simulink model "gm_sampleModel1512_5_sub"  (R2023a)
settings: Solver=VariableStepAuto  StartTime=0.0  StopTime=10.0  RelTol=1e-3
libraries: simulink x2
settings Model: Creator=user1  LastModifiedBy=user1
settings OptimizationCC: BlockReduction=off  ConditionallyExecuteInputs=off
settings DebuggingCC: InheritedTsInSrcMsg=none

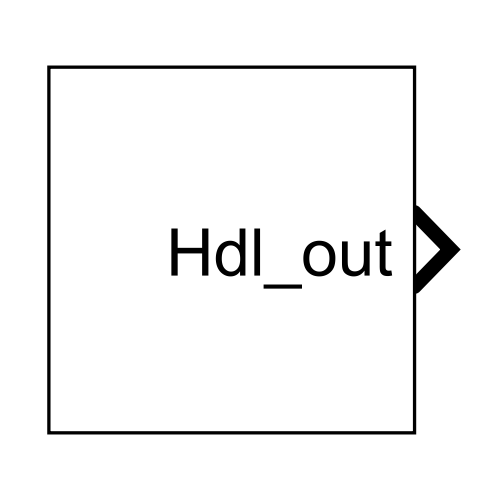
[thumbnail: Simulink's stored preview of the top-level diagram]
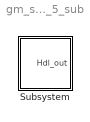
== system gm_sampleModel1512_5_sub ==
  Subsystem : Subsystem

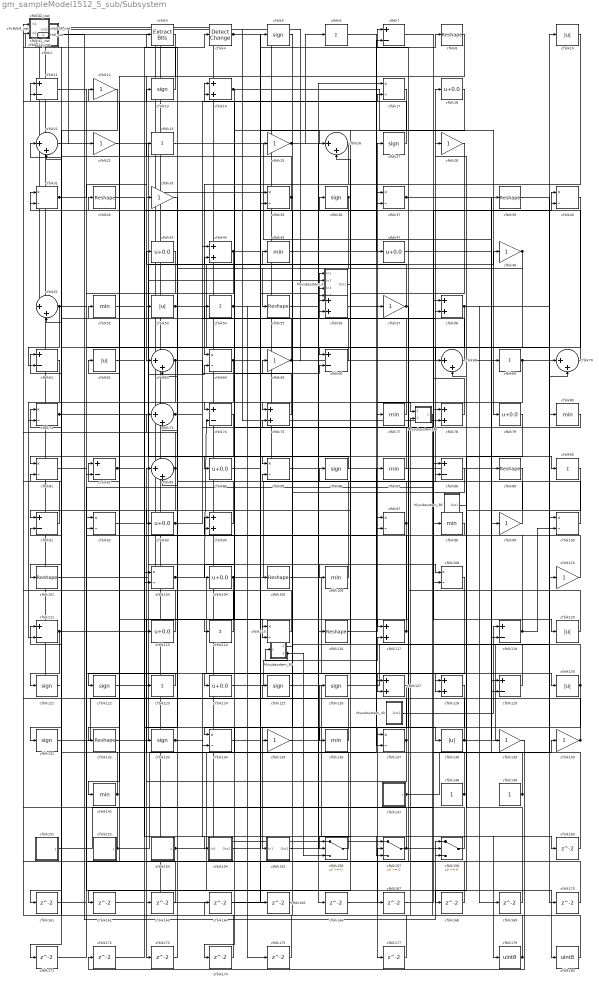
== system gm_sampleModel1512_5_sub/Subsystem ==
  Mysubsystem_3 : Subsystem
  Mysubsystem_30 : Subsystem
  Mysubsystem_36 : Subsystem
  Mysubsystem_38 : Subsystem
  Mysubsystem_40 : Subsystem
  cfblk1 : Subsystem  mask(Detect Rise Nonnegative){vinit=double(0), InputProcessing=Elements as channels (sample based), OutDataTypeStr=uint8}
      mask prompts: vinit "Simulink:masks:InitialCondition_MP"; InputProcessing "Simulink:masks:InputProcessing_MP"; OutDataTypeStr "Simulink:masks:OutputDataType_MP"
      mask help: Simulink:masks:DetectRiseNonnegative_MD
      mask init:
      | InputProcessing = 'Elements as channels (sample based)';
      | OutDataTypeStr = 'uint8';
      | vinit = double(0);
      mask TypeOptions InputProcessing: Simulink:masks:ColumnsAsChannelsFrameBased | Simulink:masks:ElementsAsChannelsSampleBased
      mask TypeOptions OutDataTypeStr: Simulink:masks:uint8 | Simulink:masks:boolean
      mask Display: fprintf('U >= 0\n&  NOT\nU/z >= 0')
  cfblk{10,53,62,120,130,138} (6 alike) : Abs  OutDataTypeStr=uint8  SaturateOnIntegerOverflow=off
  cfblk{17,31,35,37,40,64,71,81,85,92,97,100,103,108,115,134,137} (17 alike) : Product  Inputs=*/  OutDataTypeStr=uint8  RndMeth=Zero  SaturateOnIntegerOverflow=on
  cfblk{8,32,39,55,89,101,105,116,132} (9 alike) : Reshape
  cfblk102_inst : Subsystem
  cfblk{18,43,47,79,84,93,104,113,124} (9 alike) : Bias  Bias=0.0  SaturateOnIntegerOverflow=off
  cfblk{45,52,77,80,87,98,106,136,142} (9 alike) : MinMax  OutDataTypeStr=uint8
  cfblk{7,11,61,66,74,82,88,91,111,119,129} (11 alike) : Sum  Inputs=+-  OutDataTypeStr=uint8
  cfblk{12,22,25,28,33,49,57,65,99,110,135,139..140} (13 alike) : Gain  OutDataTypeStr=uint8
  cfblk112_inst : Subsystem
  cfblk{6,23,54,69,90,114,123} (7 alike) : Sum  Inputs=+  OutDataTypeStr=uint8
  cfblk{14,44,56,58,75,78,94,117,127..128} (10 alike) : Sum  OutDataTypeStr=uint8
  cfblk{5,13,27,36,86,121..122,125..126,131,133} (11 alike) : Signum
  cfblk147 : Subsystem  mask(Counter Free-Running){NumBits=double(16), tsamp=double(-1)}
      mask prompts: NumBits "Simulink:masks:NumberOfBits_MP"; tsamp "Simulink:masks:SampleTime_MP"
      mask help: Simulink:masks:CounterFreeRunning_MD
  cfblk148 : Constant  OutDataTypeStr=uint8  SampleTime=-1
  cfblk149 : Constant  OutDataTypeStr=uint8  SampleTime=-1
  cfblk151 : Subsystem  mask(Counter Free-Running){NumBits=double(16), tsamp=double(-1)}
      mask prompts: NumBits "Simulink:masks:NumberOfBits_MP"; tsamp "Simulink:masks:SampleTime_MP"
      mask help: Simulink:masks:CounterFreeRunning_MD
  cfblk152 : Subsystem  mask(Counter Limited){uplimit=double(7), tsamp=double(-1)}
      mask prompts: uplimit "Simulink:masks:UpperLimit_MP"; tsamp "Simulink:masks:SampleTime_MP"
      mask help: Simulink:masks:CounterLimited_MD
      mask init:
      | nbits = double(8);
      | tsamp = double(-1);
      | uplimit = double(7);
  cfblk153 : Subsystem  mask(Counter Limited){uplimit=double(7), tsamp=double(-1)}
      mask prompts: uplimit "Simulink:masks:UpperLimit_MP"; tsamp "Simulink:masks:SampleTime_MP"
      mask help: Simulink:masks:CounterLimited_MD
      mask init:
      | nbits = double(8);
      | tsamp = double(-1);
      | uplimit = double(7);
  cfblk154 : Subsystem
  cfblk155 : Subsystem
  cfblk156 : Switch  OutDataTypeStr=uint8  SaturateOnIntegerOverflow=off  InputSameDT=off
  cfblk157 : Switch  OutDataTypeStr=uint8  SaturateOnIntegerOverflow=off  InputSameDT=off
  cfblk158 : Switch  OutDataTypeStr=uint8  SaturateOnIntegerOverflow=off  InputSameDT=off
  cfblk{160..175,177} (17 alike) : Delay  SampleTime=1
  cfblk179 : DataTypeConversion  OutDataTypeStr=uint8  SaturateOnIntegerOverflow=off  RndMeth=Floor
  cfblk180 : DataTypeConversion  OutDataTypeStr=uint8  SaturateOnIntegerOverflow=off  RndMeth=Floor
  cfblk2 : Constant  Value=0  OutDataTypeStr=uint8  SampleTime=1
  cfblk{21,26,51,63,68,70,73,83} (8 alike) : Sum  Inputs=|++  OutDataTypeStr=uint8
  cfblk3 : simulink/Logic and Bit Operations/Extract Bits  bitsToExtract=Upper half  numBits=8  bitIdxRange=[0 7]  outScalingMode=Preserve fixed-point scaling
      settings: LibrarySourceBlock=|
      | hdlsllib/Logic and Bit
      | Operations/Extract Bits
  cfblk4 : simulink/Logic and Bit Operations/Detect Change  vinit=0  OutDataTypeStr=uint8
      settings: LibrarySourceBlock=|
      | hdlsllib/Logic and Bit
      | Operations/Detect
      | Change
  cfblk41_inst : Subsystem
  cfblk42_inst : Subsystem
  cfblk59_inst : Subsystem
  cfblk9_inst : Subsystem
  Hdl_out : Outport  OutDataTypeStr=uint8  SampleTime=1
  wires:
  Mysubsystem_3/1(Out1) -> cfblk162/1
  Mysubsystem_30/1(Out1) -> cfblk85/2
  Mysubsystem_30/2(Out2) -> cfblk156/3, cfblk65/1, Mysubsystem_30/1(In1)
  Mysubsystem_36/1(Out1) -> cfblk164/1
  Mysubsystem_38/1(Out1) -> cfblk134/1
  Mysubsystem_40/1(Out1) -> cfblk119/1
  cfblk1/1(Y) -> cfblk158/1
  cfblk10/1 -> cfblk64/1
  cfblk100/1 -> cfblk86/1
  cfblk101/1 -> cfblk108/1
  cfblk102_inst/1(out1) -> cfblk22/1
  cfblk103/1 -> cfblk74/2, cfblk130/1
  cfblk104/1 -> cfblk18/1, cfblk173/1
  cfblk105/1 -> cfblk127/2
  cfblk106/1 -> cfblk42_inst/2(in2)
  cfblk108/1 -> cfblk134/2
  cfblk11/1 -> cfblk92/2
  cfblk110/1 -> Mysubsystem_3/1(In1)
  cfblk111/1 -> cfblk121/1, Mysubsystem_3/2(In2)
  cfblk112_inst/1(out1) -> cfblk9_inst/2(in2), cfblk89/1, cfblk78/2
  cfblk113/1 -> cfblk62/1
  cfblk114/1 -> cfblk102_inst/1(in1)
  cfblk115/1 -> cfblk12/1
  cfblk116/1 -> cfblk27/1
  cfblk117/1 -> cfblk26/2, cfblk77/1
  cfblk119/1 -> cfblk28/1, cfblk100/2
  cfblk12/1 -> cfblk131/1
  cfblk120/1 -> cfblk37/2
  cfblk121/1 -> Hdl_out/1
  cfblk122/1 -> cfblk47/1
  cfblk123/1 -> cfblk122/1
  cfblk124/1 -> cfblk117/2
  cfblk125/1 -> cfblk179/1
  cfblk126/1 -> cfblk80/1
  cfblk127/1 -> cfblk177/1
  cfblk128/1 -> cfblk155/1(In1)
  cfblk129/1 -> cfblk32/1
  cfblk13/1 -> cfblk112_inst/2(in2)
  cfblk130/1 -> cfblk36/1, cfblk174/1, cfblk168/1
  cfblk131/1 -> Mysubsystem_3/3(In3)
  cfblk132/1 -> cfblk64/2
  cfblk133/1 -> cfblk83/2, cfblk156/2
  cfblk134/1 -> cfblk165/1
  cfblk135/1 -> cfblk126/1
  cfblk136/1 -> cfblk71/1
  cfblk137/1 -> cfblk51/2, cfblk163/1
  cfblk138/1 -> cfblk70/2, cfblk45/1
  cfblk139/1 -> cfblk172/1
  cfblk14/1 -> cfblk79/1, cfblk74/1
  cfblk140/1 -> cfblk9_inst/1(in1), cfblk88/2
  cfblk142/1 -> cfblk21/1, cfblk81/2
  cfblk147/1(y) -> cfblk39/1, cfblk10/1
  cfblk148/1 -> cfblk94/1, cfblk83/1
  cfblk149/1 -> cfblk94/2, cfblk61/1
  cfblk151/1(y) -> cfblk98/1
  cfblk152/1(y) -> cfblk5/1, cfblk111/1
  cfblk153/1(y) -> cfblk180/1, cfblk87/1
  cfblk154/1(Out1) -> cfblk56/1
  cfblk155/1(Out1) -> Mysubsystem_3/4(In4)
  cfblk156/1 -> cfblk52/1
  cfblk157/1 -> cfblk102_inst/2(in2), cfblk140/1
  cfblk158/1 -> cfblk97/2
  cfblk160/1 -> cfblk44/2
  cfblk161/1 -> cfblk158/3
  cfblk162/1 -> cfblk97/1
  cfblk163/1 -> cfblk82/1
  cfblk164/1 -> cfblk158/2
  cfblk165/1 -> cfblk1/1(U)
  cfblk166/1 -> cfblk157/2
  cfblk167/1 -> cfblk40/1
  cfblk168/1 -> cfblk7/1
  cfblk169/1 -> cfblk68/2
  cfblk17/1 -> cfblk104/1
  cfblk170/1 -> cfblk41_inst/2(in2)
  cfblk171/1 -> cfblk88/1
  cfblk172/1 -> cfblk37/1
  cfblk173/1 -> cfblk73/2
  cfblk174/1 -> cfblk31/1
  cfblk175/1 -> cfblk91/2
  cfblk177/1 -> cfblk59_inst/1(in1)
  cfblk179/1 -> cfblk3/1, Mysubsystem_36/2(In2)
  cfblk18/1 -> cfblk156/1
  cfblk180/1 -> cfblk125/1
  cfblk2/1 -> cfblk157/1
  cfblk21/1 -> cfblk69/1
  cfblk22/1 -> cfblk90/1
  cfblk23/1 -> cfblk139/1
  cfblk25/1 -> cfblk116/1, cfblk6/1
  cfblk26/1 -> cfblk115/2
  cfblk27/1 -> cfblk42_inst/1(in1)
  cfblk28/1 -> cfblk91/1
  cfblk3/1 -> cfblk63/1
  cfblk31/1 -> cfblk33/1, cfblk167/1
  cfblk32/1 -> cfblk154/1(In1)
  cfblk33/1 -> cfblk113/1
  cfblk35/1 -> cfblk11/1, cfblk31/2
  cfblk36/1 -> cfblk93/1, cfblk85/1
  cfblk37/1 -> cfblk129/1, cfblk40/2
  cfblk39/1 -> cfblk100/1
  cfblk4/1 -> cfblk56/2, cfblk26/1, cfblk108/2
  cfblk40/1 -> cfblk68/1
  cfblk41_inst/1(out1) -> cfblk25/1
  cfblk42_inst/1(out1) -> cfblk35/1
  cfblk43/1 -> cfblk53/1
  cfblk44/1 -> cfblk82/2, cfblk8/1
  cfblk45/1 -> cfblk7/2
  cfblk47/1 -> cfblk119/2
  cfblk49/1 -> cfblk55/1, cfblk129/2, cfblk81/1
  cfblk5/1 -> cfblk75/1
  cfblk51/1 -> cfblk61/2, cfblk128/2
  cfblk52/1 -> cfblk66/1
  cfblk53/1 -> cfblk49/1, cfblk110/1
  cfblk54/1 -> cfblk35/2, cfblk175/1
  cfblk55/1 -> cfblk57/1
  cfblk56/1 -> Mysubsystem_36/1(In1)
  cfblk57/1 -> cfblk13/1, cfblk137/1
  cfblk58/1 -> cfblk63/2, cfblk170/1, cfblk169/1, cfblk114/1
  cfblk59_inst/1(out1) -> cfblk51/1, cfblk105/1
  cfblk6/1 -> cfblk138/1
  cfblk61/1 -> cfblk111/2
  cfblk62/1 -> cfblk103/1
  cfblk63/1 -> cfblk66/2, cfblk171/1
  cfblk64/1 -> cfblk161/1, cfblk160/1
  cfblk65/1 -> cfblk157/3, cfblk112_inst/1(in1)
  cfblk66/1 -> cfblk23/1
  cfblk68/1 -> cfblk44/1
  cfblk69/1 -> cfblk117/1, cfblk71/2
  cfblk7/1 -> cfblk120/1
  cfblk70/1 -> cfblk21/2
  cfblk71/1 -> cfblk99/1, cfblk166/1
  cfblk73/1 -> cfblk58/2, cfblk133/1
  cfblk74/1 -> cfblk101/1
  cfblk75/1 -> cfblk54/1
  cfblk77/1 -> cfblk11/2
  cfblk78/1 -> cfblk58/1
  cfblk79/1 -> cfblk128/1
  cfblk8/1 -> cfblk132/1
  cfblk80/1 -> cfblk75/2
  cfblk81/1 -> cfblk124/1
  cfblk82/1 -> cfblk137/2, cfblk115/1
  cfblk83/1 -> cfblk59_inst/2(in2), cfblk103/2, cfblk123/1
  cfblk84/1 -> cfblk106/1
  cfblk85/1 -> cfblk17/1
  cfblk86/1 -> cfblk84/1
  cfblk87/1 -> cfblk14/1
  cfblk88/1 -> cfblk135/1
  cfblk89/1 -> cfblk127/1
  cfblk9_inst/1(out1) -> cfblk70/1
  cfblk90/1 -> cfblk136/1
  cfblk91/1 -> cfblk41_inst/1(in1)
  cfblk92/1 -> cfblk4/1
  cfblk93/1 -> cfblk78/1, cfblk17/2
  cfblk94/1 -> cfblk43/1
  cfblk97/1 -> cfblk73/1, cfblk142/1
  cfblk98/1 -> cfblk92/1
  cfblk99/1 -> cfblk14/2

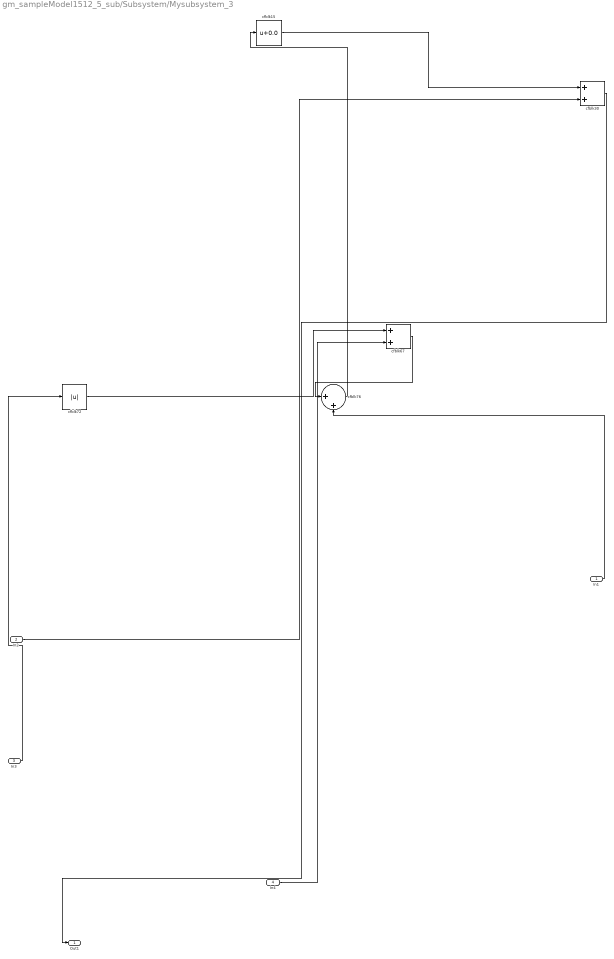
== system gm_sampleModel1512_5_sub/Subsystem/Mysubsystem_3 ==
  In1 : Inport  OutDataTypeStr=uint8  PortDimensions=1  SampleTime=1
  In2 : Inport  Port=2  OutDataTypeStr=uint8  PortDimensions=1  SampleTime=1
  In3 : Inport  Port=3  OutDataTypeStr=uint8  PortDimensions=1  SampleTime=1
  In4 : Inport  Port=4  OutDataTypeStr=uint8  PortDimensions=1  SampleTime=1
  cfblk15 : Bias  Bias=0.0  SaturateOnIntegerOverflow=off
  cfblk30 : Sum
  cfblk67 : Sum
  cfblk72 : Abs  SaturateOnIntegerOverflow=off
  cfblk76 : Sum  Inputs=|++
  Out1 : Outport  SampleTime=1
  wires:
  In1/1 -> cfblk76/2
  In2/1 -> cfblk30/2
  In3/1 -> cfblk72/1
  In4/1 -> cfblk67/2
  cfblk15/1 -> cfblk30/1
  cfblk30/1 -> Out1/1
  cfblk67/1 -> cfblk76/1
  cfblk72/1 -> cfblk67/1
  cfblk76/1 -> cfblk15/1

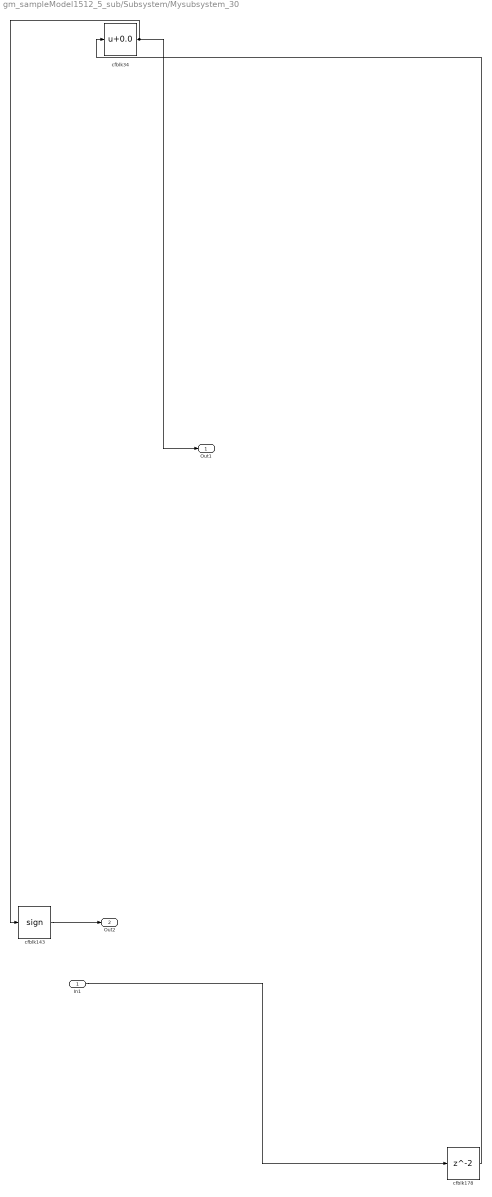
== system gm_sampleModel1512_5_sub/Subsystem/Mysubsystem_30 ==
  In1 : Inport  OutDataTypeStr=uint8  PortDimensions=1  SampleTime=1
  cfblk143 : Signum
  cfblk178 : Delay  SampleTime=1
  cfblk34 : Bias  Bias=0.0  SaturateOnIntegerOverflow=off
  Out1 : Outport  SampleTime=1
  Out2 : Outport  Port=2  SampleTime=1
  wires:
  In1/1 -> cfblk178/1
  cfblk143/1 -> Out2/1
  cfblk178/1 -> cfblk34/1
  cfblk34/1 -> cfblk143/1, Out1/1

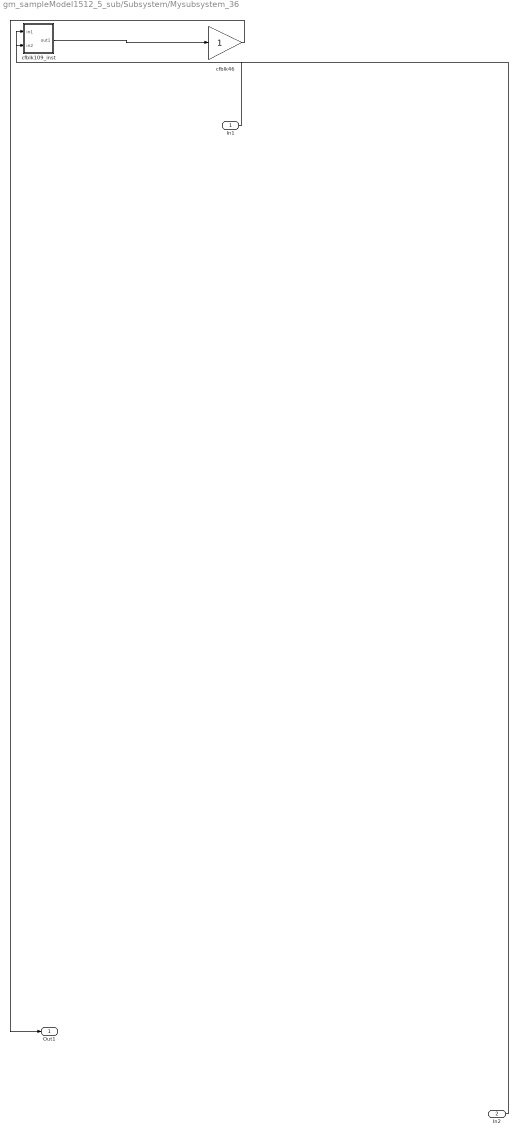
== system gm_sampleModel1512_5_sub/Subsystem/Mysubsystem_36 ==
  In1 : Inport  OutDataTypeStr=uint8  PortDimensions=1  SampleTime=1
  In2 : Inport  Port=2  OutDataTypeStr=uint8  PortDimensions=1  SampleTime=1
  cfblk109_inst : Subsystem
  cfblk46 : Gain
  Out1 : Outport  SampleTime=1
  wires:
  In1/1 -> cfblk109_inst/1(in1)
  In2/1 -> cfblk109_inst/2(in2)
  cfblk109_inst/1(out1) -> cfblk46/1
  cfblk46/1 -> Out1/1

== system gm_sampleModel1512_5_sub/Subsystem/Mysubsystem_38 ==
  cfblk150 : Subsystem  mask(Counter Limited){uplimit=double(7), tsamp=double(-1)}
      mask prompts: uplimit "Simulink:masks:UpperLimit_MP"; tsamp "Simulink:masks:SampleTime_MP"
      mask help: Simulink:masks:CounterLimited_MD
      mask init:
      | nbits = double(8);
      | tsamp = double(-1);
      | uplimit = double(7);
  cfblk38 : Sum  Inputs=+
  cfblk96 : Reshape
  Out1 : Outport  SampleTime=1
  wires:
  cfblk150/1(y) -> cfblk96/1
  cfblk38/1 -> Out1/1
  cfblk96/1 -> cfblk38/1

== system gm_sampleModel1512_5_sub/Subsystem/Mysubsystem_40 ==
  cfblk118 : Signum
  cfblk146 : Subsystem  mask(Counter Free-Running){NumBits=double(16), tsamp=double(-1)}
      mask prompts: NumBits "Simulink:masks:NumberOfBits_MP"; tsamp "Simulink:masks:SampleTime_MP"
      mask help: Simulink:masks:CounterFreeRunning_MD
  Out1 : Outport  SampleTime=1
  wires:
  cfblk118/1 -> Out1/1
  cfblk146/1(y) -> cfblk118/1

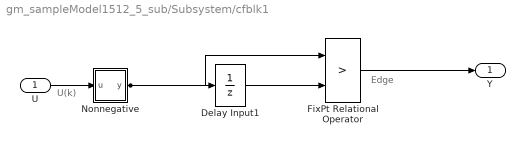
== system gm_sampleModel1512_5_sub/Subsystem/cfblk1 ==
  note: U(k)
  note: Edge
  U : Inport  OutDataTypeStr=uint8  SampleTime=1
  Delay Input1 : UnitDelay  Description=Store in Global RAM  DisableCoverage=on  InitialCondition=vinit  SampleTime=-1  HasFrameUpgradeWarning=on
  FixPt Relational Operator : RelationalOperator  Operator=>  OutDataTypeStr=fixdt(0, 8)  ZeroCross=off  InputSameDT=off
  Nonnegative : Subsystem  mask(Compare To Zero){relop=>=, OutDataTypeStr=boolean, ZeroCross=off}
      mask prompts: relop "Simulink:masks:Operator_MP"; OutDataTypeStr "Simulink:masks:OutputDataType_MP"; ZeroCross "Simulink:masks:EnableZerocrossingDetection_MP"
      mask help: Simulink:masks:CompareToZero_MD
      mask init:
      | OutDataTypeStr = 'boolean';
      | ZeroCross = 'off';
      | blkName = 'sampleModel1512_5_sub/Subsystem/cfblk1/Nonnegative';
      | relop = '>=';
      | setValue = 'boolean';
      mask TypeOptions relop: == | ~= | < | <= | >= | >
      mask TypeOptions OutDataTypeStr: Simulink:masks:uint8 | Simulink:masks:boolean
      mask Callback ZeroCross: sl('zeroCrossEnable', gcbh);
      mask Display: disp([relop,' 0'])
  Y : Outport  SampleTime=1
  wires:
  U/1 -> Nonnegative/1(u)
  Delay Input1/1 -> FixPt Relational Operator/2
  FixPt Relational Operator/1 -> Y/1
  Nonnegative/1(y) -> FixPt Relational Operator/1, Delay Input1/1

== system gm_sampleModel1512_5_sub/Subsystem/cfblk102_inst ==
  in1 : Inport  OutDataTypeStr=uint8  SampleTime=1
  in2 : Inport  Port=2  OutDataTypeStr=uint8  SampleTime=1
  mul_cfblk102_dotp_mulcomp : Product  Inputs=**  OutDataTypeStr=uint8  SampleTime=1
  out1 : Outport  OutDataTypeStr=uint8  SampleTime=1
  wires:
  in1/1 -> mul_cfblk102_dotp_mulcomp/1
  in2/1 -> mul_cfblk102_dotp_mulcomp/2
  mul_cfblk102_dotp_mulcomp/1 -> out1/1

== system gm_sampleModel1512_5_sub/Subsystem/cfblk112_inst ==
  in1 : Inport  OutDataTypeStr=uint8  SampleTime=1
  in2 : Inport  Port=2  OutDataTypeStr=uint8  SampleTime=1
  mul_cfblk112_dotp_mulcomp : Product  Inputs=**  OutDataTypeStr=uint8  SampleTime=1
  out1 : Outport  OutDataTypeStr=uint8  SampleTime=1
  wires:
  in1/1 -> mul_cfblk112_dotp_mulcomp/1
  in2/1 -> mul_cfblk112_dotp_mulcomp/2
  mul_cfblk112_dotp_mulcomp/1 -> out1/1

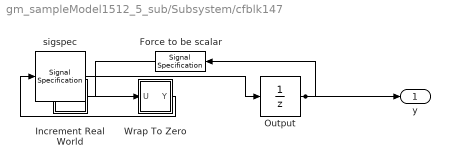
== system gm_sampleModel1512_5_sub/Subsystem/cfblk147 ==
  Force to be scalar : SignalSpecification  DisableCoverage=on  Dimensions=1
  Increment Real World : Subsystem  mask(Real World Value Increment){}
      mask help: Simulink:masks:RealWorldValueIncrement_MD
      mask Display: disp('V++')
  Output : UnitDelay  InitialCondition=0.0  SampleTime=tsamp  HasFrameUpgradeWarning=on
  Wrap To Zero : Subsystem  mask(Wrap To Zero){Threshold=double(65535)}
      mask prompts: Threshold "Simulink:masks:Threshold_MP"
      mask help: Simulink:masks:WrapToZero_MD
  sigspec : SignalSpecification  OutDataTypeStr=uint16  Dimensions=1
  y : Outport  SampleTime=1
  wires:
  Force to be scalar/1 -> Increment Real World/1(u)
  Increment Real World/1(y) -> Wrap To Zero/1(U)
  Output/1 -> Force to be scalar/1, y/1
  Wrap To Zero/1(Y) -> sigspec/1
  sigspec/1 -> Output/1

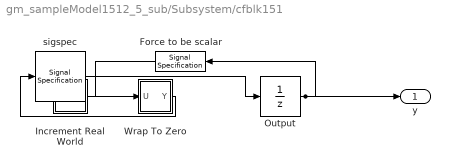
== system gm_sampleModel1512_5_sub/Subsystem/cfblk151 ==
  Force to be scalar : SignalSpecification  DisableCoverage=on  Dimensions=1
  Increment Real World : Subsystem  mask(Real World Value Increment){}
      mask help: Simulink:masks:RealWorldValueIncrement_MD
      mask Display: disp('V++')
  Output : UnitDelay  InitialCondition=0.0  SampleTime=tsamp  HasFrameUpgradeWarning=on
  Wrap To Zero : Subsystem  mask(Wrap To Zero){Threshold=double(65535)}
      mask prompts: Threshold "Simulink:masks:Threshold_MP"
      mask help: Simulink:masks:WrapToZero_MD
  sigspec : SignalSpecification  OutDataTypeStr=uint16  Dimensions=1
  y : Outport  SampleTime=1
  wires:
  Force to be scalar/1 -> Increment Real World/1(u)
  Increment Real World/1(y) -> Wrap To Zero/1(U)
  Output/1 -> Force to be scalar/1, y/1
  Wrap To Zero/1(Y) -> sigspec/1
  sigspec/1 -> Output/1

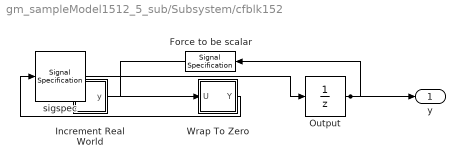
== system gm_sampleModel1512_5_sub/Subsystem/cfblk152 ==
  Force to be scalar : SignalSpecification  DisableCoverage=on  Dimensions=1
  Increment Real World : Subsystem  mask(Real World Value Increment){}
      mask help: Simulink:masks:RealWorldValueIncrement_MD
      mask Display: disp('V++')
  Output : UnitDelay  InitialCondition=0.0  SampleTime=tsamp  HasFrameUpgradeWarning=on
  Wrap To Zero : Subsystem  mask(Wrap To Zero){Threshold=double(7)}
      mask prompts: Threshold "Simulink:masks:Threshold_MP"
      mask help: Simulink:masks:WrapToZero_MD
  sigspec : SignalSpecification  OutDataTypeStr=uint8  Dimensions=1
  y : Outport  SampleTime=1
  wires:
  Force to be scalar/1 -> Increment Real World/1(u)
  Increment Real World/1(y) -> Wrap To Zero/1(U)
  Output/1 -> Force to be scalar/1, y/1
  Wrap To Zero/1(Y) -> sigspec/1
  sigspec/1 -> Output/1

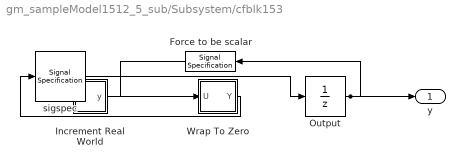
== system gm_sampleModel1512_5_sub/Subsystem/cfblk153 ==
  Force to be scalar : SignalSpecification  DisableCoverage=on  Dimensions=1
  Increment Real World : Subsystem  mask(Real World Value Increment){}
      mask help: Simulink:masks:RealWorldValueIncrement_MD
      mask Display: disp('V++')
  Output : UnitDelay  InitialCondition=0.0  SampleTime=tsamp  HasFrameUpgradeWarning=on
  Wrap To Zero : Subsystem  mask(Wrap To Zero){Threshold=double(7)}
      mask prompts: Threshold "Simulink:masks:Threshold_MP"
      mask help: Simulink:masks:WrapToZero_MD
  sigspec : SignalSpecification  OutDataTypeStr=uint8  Dimensions=1
  y : Outport  SampleTime=1
  wires:
  Force to be scalar/1 -> Increment Real World/1(u)
  Increment Real World/1(y) -> Wrap To Zero/1(U)
  Output/1 -> Force to be scalar/1, y/1
  Wrap To Zero/1(Y) -> sigspec/1
  sigspec/1 -> Output/1

== system gm_sampleModel1512_5_sub/Subsystem/cfblk154 ==
  In1 : Inport  OutDataTypeStr=uint8  PortDimensions=1  SampleTime=1
  Out1 : Outport  SampleTime=1
  wires:
  In1/1 -> Out1/1

== system gm_sampleModel1512_5_sub/Subsystem/cfblk155 ==
  In1 : Inport  OutDataTypeStr=uint8  PortDimensions=1  SampleTime=1
  Out1 : Outport  SampleTime=1
  wires:
  In1/1 -> Out1/1

== system gm_sampleModel1512_5_sub/Subsystem/cfblk41_inst ==
  in1 : Inport  OutDataTypeStr=uint8  SampleTime=1
  in2 : Inport  Port=2  OutDataTypeStr=uint8  SampleTime=1
  mul_cfblk41_dotp_mulcomp : Product  Inputs=**  OutDataTypeStr=uint8  SampleTime=1
  out1 : Outport  OutDataTypeStr=uint8  SampleTime=1
  wires:
  in1/1 -> mul_cfblk41_dotp_mulcomp/1
  in2/1 -> mul_cfblk41_dotp_mulcomp/2
  mul_cfblk41_dotp_mulcomp/1 -> out1/1

== system gm_sampleModel1512_5_sub/Subsystem/cfblk42_inst ==
  in1 : Inport  OutDataTypeStr=uint8  SampleTime=1
  in2 : Inport  Port=2  OutDataTypeStr=uint8  SampleTime=1
  mul_cfblk42_dotp_mulcomp : Product  Inputs=**  OutDataTypeStr=uint8  SampleTime=1
  out1 : Outport  OutDataTypeStr=uint8  SampleTime=1
  wires:
  in1/1 -> mul_cfblk42_dotp_mulcomp/1
  in2/1 -> mul_cfblk42_dotp_mulcomp/2
  mul_cfblk42_dotp_mulcomp/1 -> out1/1

== system gm_sampleModel1512_5_sub/Subsystem/cfblk59_inst ==
  in1 : Inport  OutDataTypeStr=uint8  SampleTime=1
  in2 : Inport  Port=2  OutDataTypeStr=uint8  SampleTime=1
  mul_cfblk59_dotp_mulcomp : Product  Inputs=**  OutDataTypeStr=uint8  SampleTime=1
  out1 : Outport  OutDataTypeStr=uint8  SampleTime=1
  wires:
  in1/1 -> mul_cfblk59_dotp_mulcomp/1
  in2/1 -> mul_cfblk59_dotp_mulcomp/2
  mul_cfblk59_dotp_mulcomp/1 -> out1/1

== system gm_sampleModel1512_5_sub/Subsystem/cfblk9_inst ==
  in1 : Inport  OutDataTypeStr=uint8  SampleTime=1
  in2 : Inport  Port=2  OutDataTypeStr=uint8  SampleTime=1
  mul_cfblk9_dotp_mulcomp : Product  Inputs=**  OutDataTypeStr=uint8  SampleTime=1
  out1 : Outport  OutDataTypeStr=uint8  SampleTime=1
  wires:
  in1/1 -> mul_cfblk9_dotp_mulcomp/1
  in2/1 -> mul_cfblk9_dotp_mulcomp/2
  mul_cfblk9_dotp_mulcomp/1 -> out1/1

== system gm_sampleModel1512_5_sub/Subsystem/Mysubsystem_36/cfblk109_inst ==
  in1 : Inport  OutDataTypeStr=uint8  SampleTime=1
  in2 : Inport  Port=2  OutDataTypeStr=uint8  SampleTime=1
  mul_cfblk109_dotp_mulcomp : Product  Inputs=**  OutDataTypeStr=uint16  SampleTime=1
  out1 : Outport  OutDataTypeStr=uint16  SampleTime=1
  wires:
  in1/1 -> mul_cfblk109_dotp_mulcomp/1
  in2/1 -> mul_cfblk109_dotp_mulcomp/2
  mul_cfblk109_dotp_mulcomp/1 -> out1/1

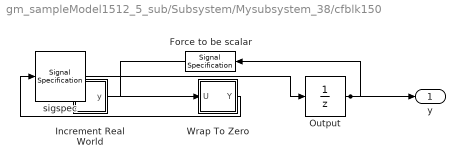
== system gm_sampleModel1512_5_sub/Subsystem/Mysubsystem_38/cfblk150 ==
  Force to be scalar : SignalSpecification  DisableCoverage=on  Dimensions=1
  Increment Real World : Subsystem  mask(Real World Value Increment){}
      mask help: Simulink:masks:RealWorldValueIncrement_MD
      mask Display: disp('V++')
  Output : UnitDelay  InitialCondition=0.0  SampleTime=tsamp  HasFrameUpgradeWarning=on
  Wrap To Zero : Subsystem  mask(Wrap To Zero){Threshold=double(7)}
      mask prompts: Threshold "Simulink:masks:Threshold_MP"
      mask help: Simulink:masks:WrapToZero_MD
  sigspec : SignalSpecification  OutDataTypeStr=uint8  Dimensions=1
  y : Outport  SampleTime=1
  wires:
  Force to be scalar/1 -> Increment Real World/1(u)
  Increment Real World/1(y) -> Wrap To Zero/1(U)
  Output/1 -> Force to be scalar/1, y/1
  Wrap To Zero/1(Y) -> sigspec/1
  sigspec/1 -> Output/1

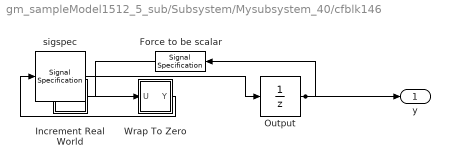
== system gm_sampleModel1512_5_sub/Subsystem/Mysubsystem_40/cfblk146 ==
  Force to be scalar : SignalSpecification  DisableCoverage=on  Dimensions=1
  Increment Real World : Subsystem  mask(Real World Value Increment){}
      mask help: Simulink:masks:RealWorldValueIncrement_MD
      mask Display: disp('V++')
  Output : UnitDelay  InitialCondition=0.0  SampleTime=tsamp  HasFrameUpgradeWarning=on
  Wrap To Zero : Subsystem  mask(Wrap To Zero){Threshold=double(65535)}
      mask prompts: Threshold "Simulink:masks:Threshold_MP"
      mask help: Simulink:masks:WrapToZero_MD
  sigspec : SignalSpecification  OutDataTypeStr=uint16  Dimensions=1
  y : Outport  SampleTime=1
  wires:
  Force to be scalar/1 -> Increment Real World/1(u)
  Increment Real World/1(y) -> Wrap To Zero/1(U)
  Output/1 -> Force to be scalar/1, y/1
  Wrap To Zero/1(Y) -> sigspec/1
  sigspec/1 -> Output/1

== system gm_sampleModel1512_5_sub/Subsystem/cfblk1/Nonnegative ==
  u : Inport  OutDataTypeStr=uint8  SampleTime=1
  Compare : RelationalOperator  OutDataTypeStr=boolean  ZeroCross=off
  Constant : Constant  DisableCoverage=on  Value=0  OutDataTypeStr=Inherit: Inherit via back propagation  SampleTime=-1  PreserveConstantTs=on
  y : Outport  SampleTime=1
  wires:
  u/1 -> Compare/1
  Compare/1 -> y/1
  Constant/1 -> Compare/2

== system gm_sampleModel1512_5_sub/Subsystem/cfblk147/Increment Real World ==
  u : Inport  OutDataTypeStr=uint16  SampleTime=1
  FixPt Constant : Constant  DisableCoverage=on  OutDataTypeStr=Inherit: Inherit via back propagation  SampleTime=-1
  FixPt Data Type Duplicate : DataTypeDuplicate  DisableCoverage=on  NumInputPorts=3
  FixPt Sum1 : Sum  InputSameDT=on  OutDataTypeStr=Inherit: Inherit via back propagation  LockScale=on
  y : Outport  SampleTime=1
  wires:
  u/1 -> FixPt Sum1/1, FixPt Data Type Duplicate/2
  FixPt Constant/1 -> FixPt Sum1/2, FixPt Data Type Duplicate/3
  FixPt Sum1/1 -> FixPt Data Type Duplicate/1, y/1

== system gm_sampleModel1512_5_sub/Subsystem/cfblk147/Wrap To Zero ==
  note: U(k)
  U : Inport  OutDataTypeStr=uint16  SampleTime=1
  Constant : Constant  DisableCoverage=on  Value=0  OutDataTypeStr=Inherit: Inherit via back propagation  SampleTime=-1
  FixPt Data Type Duplicate1 : DataTypeDuplicate  DisableCoverage=on  NumInputPorts=3
  FixPt Switch : Switch  Criteria=u2 > Threshold  Threshold=Threshold  OutDataTypeStr=Inherit: Inherit via back propagation  ZeroCross=off  SaturateOnIntegerOverflow=off  InputSameDT=off
  Y : Outport  SampleTime=1
  wires:
  U/1 -> FixPt Switch/3, FixPt Switch/2, FixPt Data Type Duplicate1/2
  Constant/1 -> FixPt Switch/1, FixPt Data Type Duplicate1/3
  FixPt Switch/1 -> FixPt Data Type Duplicate1/1, Y/1

== system gm_sampleModel1512_5_sub/Subsystem/cfblk151/Increment Real World ==
  u : Inport  OutDataTypeStr=uint16  SampleTime=1
  FixPt Constant : Constant  DisableCoverage=on  OutDataTypeStr=Inherit: Inherit via back propagation  SampleTime=-1
  FixPt Data Type Duplicate : DataTypeDuplicate  DisableCoverage=on  NumInputPorts=3
  FixPt Sum1 : Sum  InputSameDT=on  OutDataTypeStr=Inherit: Inherit via back propagation  LockScale=on
  y : Outport  SampleTime=1
  wires:
  u/1 -> FixPt Sum1/1, FixPt Data Type Duplicate/2
  FixPt Constant/1 -> FixPt Sum1/2, FixPt Data Type Duplicate/3
  FixPt Sum1/1 -> FixPt Data Type Duplicate/1, y/1

== system gm_sampleModel1512_5_sub/Subsystem/cfblk151/Wrap To Zero ==
  note: U(k)
  U : Inport  OutDataTypeStr=uint16  SampleTime=1
  Constant : Constant  DisableCoverage=on  Value=0  OutDataTypeStr=Inherit: Inherit via back propagation  SampleTime=-1
  FixPt Data Type Duplicate1 : DataTypeDuplicate  DisableCoverage=on  NumInputPorts=3
  FixPt Switch : Switch  Criteria=u2 > Threshold  Threshold=Threshold  OutDataTypeStr=Inherit: Inherit via back propagation  ZeroCross=off  SaturateOnIntegerOverflow=off  InputSameDT=off
  Y : Outport  SampleTime=1
  wires:
  U/1 -> FixPt Switch/3, FixPt Switch/2, FixPt Data Type Duplicate1/2
  Constant/1 -> FixPt Switch/1, FixPt Data Type Duplicate1/3
  FixPt Switch/1 -> FixPt Data Type Duplicate1/1, Y/1

== system gm_sampleModel1512_5_sub/Subsystem/cfblk152/Increment Real World ==
  u : Inport  OutDataTypeStr=uint8  SampleTime=1
  FixPt Constant : Constant  DisableCoverage=on  OutDataTypeStr=Inherit: Inherit via back propagation  SampleTime=-1
  FixPt Data Type Duplicate : DataTypeDuplicate  DisableCoverage=on  NumInputPorts=3
  FixPt Sum1 : Sum  InputSameDT=on  OutDataTypeStr=Inherit: Inherit via back propagation  LockScale=on
  y : Outport  SampleTime=1
  wires:
  u/1 -> FixPt Sum1/1, FixPt Data Type Duplicate/2
  FixPt Constant/1 -> FixPt Sum1/2, FixPt Data Type Duplicate/3
  FixPt Sum1/1 -> FixPt Data Type Duplicate/1, y/1

== system gm_sampleModel1512_5_sub/Subsystem/cfblk152/Wrap To Zero ==
  note: U(k)
  U : Inport  OutDataTypeStr=uint8  SampleTime=1
  Constant : Constant  DisableCoverage=on  Value=0  OutDataTypeStr=Inherit: Inherit via back propagation  SampleTime=-1
  FixPt Data Type Duplicate1 : DataTypeDuplicate  DisableCoverage=on  NumInputPorts=3
  FixPt Switch : Switch  Criteria=u2 > Threshold  Threshold=Threshold  OutDataTypeStr=Inherit: Inherit via back propagation  ZeroCross=off  SaturateOnIntegerOverflow=off  InputSameDT=off
  Y : Outport  SampleTime=1
  wires:
  U/1 -> FixPt Switch/3, FixPt Switch/2, FixPt Data Type Duplicate1/2
  Constant/1 -> FixPt Switch/1, FixPt Data Type Duplicate1/3
  FixPt Switch/1 -> FixPt Data Type Duplicate1/1, Y/1

== system gm_sampleModel1512_5_sub/Subsystem/cfblk153/Increment Real World ==
  u : Inport  OutDataTypeStr=uint8  SampleTime=1
  FixPt Constant : Constant  DisableCoverage=on  OutDataTypeStr=Inherit: Inherit via back propagation  SampleTime=-1
  FixPt Data Type Duplicate : DataTypeDuplicate  DisableCoverage=on  NumInputPorts=3
  FixPt Sum1 : Sum  InputSameDT=on  OutDataTypeStr=Inherit: Inherit via back propagation  LockScale=on
  y : Outport  SampleTime=1
  wires:
  u/1 -> FixPt Sum1/1, FixPt Data Type Duplicate/2
  FixPt Constant/1 -> FixPt Sum1/2, FixPt Data Type Duplicate/3
  FixPt Sum1/1 -> FixPt Data Type Duplicate/1, y/1

== system gm_sampleModel1512_5_sub/Subsystem/cfblk153/Wrap To Zero ==
  note: U(k)
  U : Inport  OutDataTypeStr=uint8  SampleTime=1
  Constant : Constant  DisableCoverage=on  Value=0  OutDataTypeStr=Inherit: Inherit via back propagation  SampleTime=-1
  FixPt Data Type Duplicate1 : DataTypeDuplicate  DisableCoverage=on  NumInputPorts=3
  FixPt Switch : Switch  Criteria=u2 > Threshold  Threshold=Threshold  OutDataTypeStr=Inherit: Inherit via back propagation  ZeroCross=off  SaturateOnIntegerOverflow=off  InputSameDT=off
  Y : Outport  SampleTime=1
  wires:
  U/1 -> FixPt Switch/3, FixPt Switch/2, FixPt Data Type Duplicate1/2
  Constant/1 -> FixPt Switch/1, FixPt Data Type Duplicate1/3
  FixPt Switch/1 -> FixPt Data Type Duplicate1/1, Y/1

== system gm_sampleModel1512_5_sub/Subsystem/Mysubsystem_38/cfblk150/Increment Real World ==
  u : Inport  OutDataTypeStr=uint8  SampleTime=1
  FixPt Constant : Constant  DisableCoverage=on  OutDataTypeStr=Inherit: Inherit via back propagation  SampleTime=-1
  FixPt Data Type Duplicate : DataTypeDuplicate  DisableCoverage=on  NumInputPorts=3
  FixPt Sum1 : Sum  InputSameDT=on  OutDataTypeStr=Inherit: Inherit via back propagation  LockScale=on
  y : Outport  SampleTime=1
  wires:
  u/1 -> FixPt Sum1/1, FixPt Data Type Duplicate/2
  FixPt Constant/1 -> FixPt Sum1/2, FixPt Data Type Duplicate/3
  FixPt Sum1/1 -> FixPt Data Type Duplicate/1, y/1

== system gm_sampleModel1512_5_sub/Subsystem/Mysubsystem_38/cfblk150/Wrap To Zero ==
  note: U(k)
  U : Inport  OutDataTypeStr=uint8  SampleTime=1
  Constant : Constant  DisableCoverage=on  Value=0  OutDataTypeStr=Inherit: Inherit via back propagation  SampleTime=-1
  FixPt Data Type Duplicate1 : DataTypeDuplicate  DisableCoverage=on  NumInputPorts=3
  FixPt Switch : Switch  Criteria=u2 > Threshold  Threshold=Threshold  OutDataTypeStr=Inherit: Inherit via back propagation  ZeroCross=off  SaturateOnIntegerOverflow=off  InputSameDT=off
  Y : Outport  SampleTime=1
  wires:
  U/1 -> FixPt Switch/3, FixPt Switch/2, FixPt Data Type Duplicate1/2
  Constant/1 -> FixPt Switch/1, FixPt Data Type Duplicate1/3
  FixPt Switch/1 -> FixPt Data Type Duplicate1/1, Y/1

== system gm_sampleModel1512_5_sub/Subsystem/Mysubsystem_40/cfblk146/Increment Real World ==
  u : Inport  OutDataTypeStr=uint16  SampleTime=1
  FixPt Constant : Constant  DisableCoverage=on  OutDataTypeStr=Inherit: Inherit via back propagation  SampleTime=-1
  FixPt Data Type Duplicate : DataTypeDuplicate  DisableCoverage=on  NumInputPorts=3
  FixPt Sum1 : Sum  InputSameDT=on  OutDataTypeStr=Inherit: Inherit via back propagation  LockScale=on
  y : Outport  SampleTime=1
  wires:
  u/1 -> FixPt Sum1/1, FixPt Data Type Duplicate/2
  FixPt Constant/1 -> FixPt Sum1/2, FixPt Data Type Duplicate/3
  FixPt Sum1/1 -> FixPt Data Type Duplicate/1, y/1

== system gm_sampleModel1512_5_sub/Subsystem/Mysubsystem_40/cfblk146/Wrap To Zero ==
  note: U(k)
  U : Inport  OutDataTypeStr=uint16  SampleTime=1
  Constant : Constant  DisableCoverage=on  Value=0  OutDataTypeStr=Inherit: Inherit via back propagation  SampleTime=-1
  FixPt Data Type Duplicate1 : DataTypeDuplicate  DisableCoverage=on  NumInputPorts=3
  FixPt Switch : Switch  Criteria=u2 > Threshold  Threshold=Threshold  OutDataTypeStr=Inherit: Inherit via back propagation  ZeroCross=off  SaturateOnIntegerOverflow=off  InputSameDT=off
  Y : Outport  SampleTime=1
  wires:
  U/1 -> FixPt Switch/3, FixPt Switch/2, FixPt Data Type Duplicate1/2
  Constant/1 -> FixPt Switch/1, FixPt Data Type Duplicate1/3
  FixPt Switch/1 -> FixPt Data Type Duplicate1/1, Y/1
